simulink model "steadystateerror"  (R2021b)
settings: Solver=VariableStepAuto  StartTime=0.0  StopTime=100.0  RelTol=1e-3
libraries: cstblocks x6, simulink x3
settings Model: Creator=PRANAV ARYA  LastModifiedBy=PRANAV ARYA

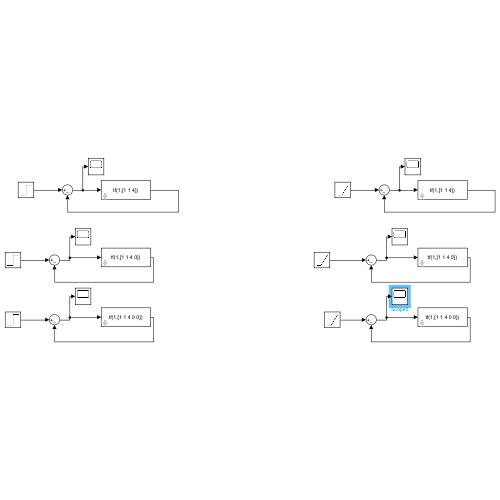
[thumbnail: Simulink's stored preview of the top-level diagram]
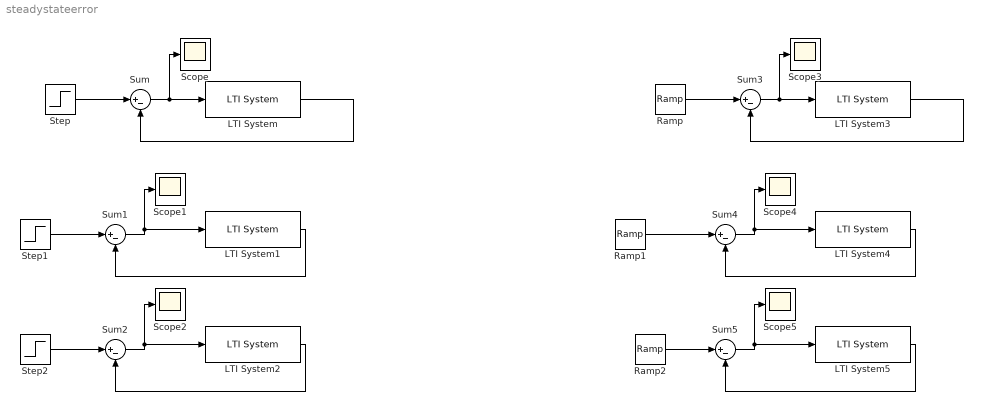
== system steadystateerror ==
  LTI System : cstblocks/LTI System  sys=tf(1,[1 1 4])  IC=[]
  LTI System1 : cstblocks/LTI System  sys=tf(1,[1 1 4 0])  IC=[]
  LTI System2 : cstblocks/LTI System  sys=tf(1,[1 1 4 0 0])  IC=[]
  LTI System3 : cstblocks/LTI System  sys=tf(1,[1 1 4])  IC=[]
  LTI System4 : cstblocks/LTI System  sys=tf(1,[1 1 4 0])  IC=[]
  LTI System5 : cstblocks/LTI System  sys=tf(1,[1 1 4 0 0])  IC=[]
  Ramp : simulink/Sources/Ramp  slope=1  start=0  InitialOutput=0
  Ramp1 : simulink/Sources/Ramp  slope=1  start=0  InitialOutput=0
  Ramp2 : simulink/Sources/Ramp  slope=1  start=0  InitialOutput=0
  Scope{,1..5} (6 alike) : Scope
  Step : Step  Time=0  SampleTime=0
  Step1 : Step  Time=0  SampleTime=0
  Step2 : Step  Time=0  SampleTime=0
  Sum{,1..5} (6 alike) : Sum  Inputs=|+-
  wires:
  Sum/1 -> Scope/1, LTI System/1
  LTI System/1 -> Sum/2
  Step/1 -> Sum/1
  LTI System1/1 -> Sum1/2
  Sum1/1 -> Scope1/1, LTI System1/1
  Step1/1 -> Sum1/1
  LTI System2/1 -> Sum2/2
  Step2/1 -> Sum2/1
  Sum2/1 -> Scope2/1, LTI System2/1
  Ramp2/1 -> Sum5/1
  LTI System5/1 -> Sum5/2
  Ramp1/1 -> Sum4/1
  LTI System4/1 -> Sum4/2
  Sum4/1 -> Scope4/1, LTI System4/1
  Sum5/1 -> Scope5/1, LTI System5/1
  LTI System3/1 -> Sum3/2
  Sum3/1 -> Scope3/1, LTI System3/1
  Ramp/1 -> Sum3/1
